simulink library "INT_AFS_VDDrftComp"  (R2016b)
settings: Solver=VariableStepAuto  StartTime=0.0  StopTime=10.0  RelTol=1e-3
settings Model: Creator=guanxiaoxing  LastModifiedBy=guanxiaoxing

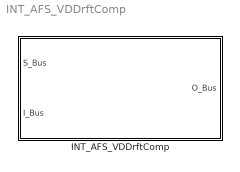
== system INT_AFS_VDDrftComp ==
  INT_AFS_VDDrftComp : Subsystem

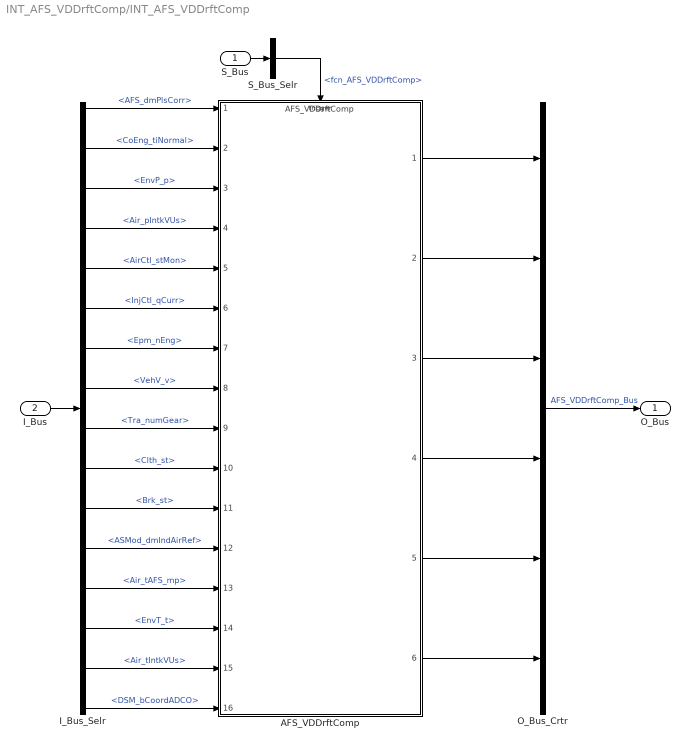
== system INT_AFS_VDDrftComp/INT_AFS_VDDrftComp ==
  S_Bus : Inport
  I_Bus : Inport  Port=2
  AFS_VDDrftComp : ModelReference  ModelNameDialog=AFS_VDDrftComp  SimulationMode=Normal  ModelReferenceVersion=1.51  TriggerPortName=function  TriggerPortTriggerType=function-call  TriggerPortStatesWhenEnabling=held
  I_Bus_Selr : BusSelector  OutputSignals=AFS_dmPlsCorr,CoEng_tiNormal,EnvP_p,Air_pIntkVUs,AirCtl_stMon,InjCtl_qCurr,Epm_nEng,VehV_v,Tra_numGear,Clth_st,Brk_st,ASMod_dmIndAirRef,Air_tAFS_mp,EnvT_t,Air_tIntkVUs,DSM_bCoordADCO
  O_Bus_Crtr : BusCreator  Inputs=6
  S_Bus_Selr : BusSelector  OutputSignals=fcn_AFS_VDDrftComp
  O_Bus : Outport
  wires:
  S_Bus_Selr/1 -> AFS_VDDrftComp/Trigger  "<fcn_AFS_VDDrftComp>"
  S_Bus/1 -> S_Bus_Selr/1
  I_Bus/1 -> I_Bus_Selr/1
  I_Bus_Selr/1 -> AFS_VDDrftComp/1  "<AFS_dmPlsCorr>"
  I_Bus_Selr/2 -> AFS_VDDrftComp/2  "<CoEng_tiNormal>"
  I_Bus_Selr/3 -> AFS_VDDrftComp/3  "<EnvP_p>"
  I_Bus_Selr/4 -> AFS_VDDrftComp/4  "<Air_pIntkVUs>"
  I_Bus_Selr/5 -> AFS_VDDrftComp/5  "<AirCtl_stMon>"
  I_Bus_Selr/6 -> AFS_VDDrftComp/6  "<InjCtl_qCurr>"
  I_Bus_Selr/7 -> AFS_VDDrftComp/7  "<Epm_nEng>"
  I_Bus_Selr/8 -> AFS_VDDrftComp/8  "<VehV_v>"
  I_Bus_Selr/9 -> AFS_VDDrftComp/9  "<Tra_numGear>"
  I_Bus_Selr/10 -> AFS_VDDrftComp/10  "<Clth_st>"
  I_Bus_Selr/11 -> AFS_VDDrftComp/11  "<Brk_st>"
  I_Bus_Selr/12 -> AFS_VDDrftComp/12  "<ASMod_dmIndAirRef>"
  I_Bus_Selr/13 -> AFS_VDDrftComp/13  "<Air_tAFS_mp>"
  I_Bus_Selr/14 -> AFS_VDDrftComp/14  "<EnvT_t>"
  I_Bus_Selr/15 -> AFS_VDDrftComp/15  "<Air_tIntkVUs>"
  I_Bus_Selr/16 -> AFS_VDDrftComp/16  "<DSM_bCoordADCO>"
  O_Bus_Crtr/1 -> O_Bus/1  "AFS_VDDrftComp_Bus"
  AFS_VDDrftComp/1 -> O_Bus_Crtr/1
  AFS_VDDrftComp/2 -> O_Bus_Crtr/2
  AFS_VDDrftComp/3 -> O_Bus_Crtr/3
  AFS_VDDrftComp/4 -> O_Bus_Crtr/4
  AFS_VDDrftComp/5 -> O_Bus_Crtr/5
  AFS_VDDrftComp/6 -> O_Bus_Crtr/6
